simulink model "egk_new1"  (Simulink 7.5)
settings: Solver=ode45  StartTime=0.0  StopTime=0.1  RelTol=1e-3
libraries: powerlib x20, powerlib_extras x2
settings Model: Creator=Administrator  LastModifiedBy=Administrator

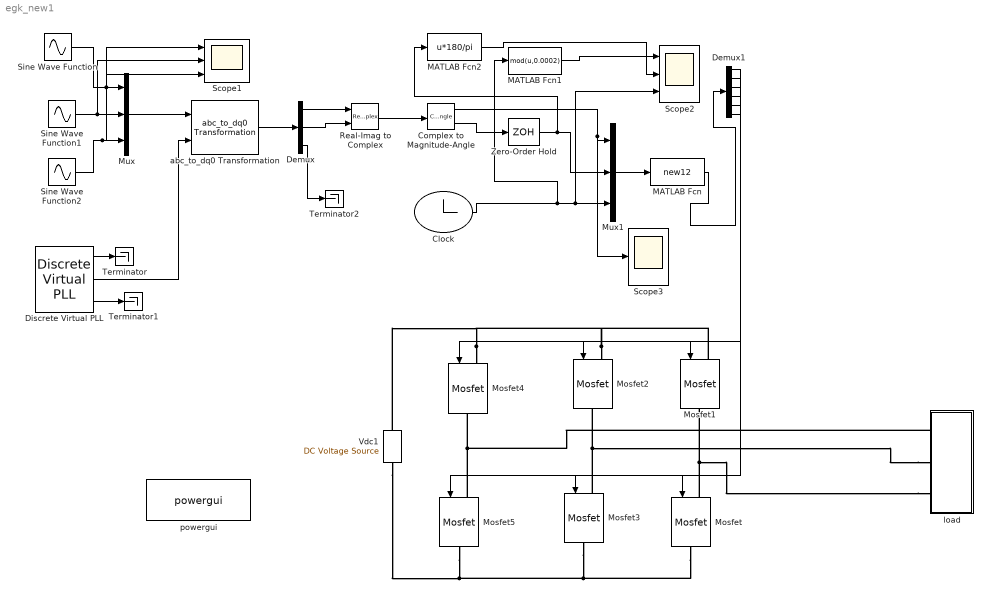
== system egk_new1 ==
  Clock : Clock
  Complex to Magnitude-Angle : ComplexToMagnitudeAngle  SampleTime=((2e-4)/8)/100
  Demux : Demux  Outputs=3
  Demux1 : Demux  Outputs=6
  Discrete Virtual PLL : powerlib_extras/Discrete  Control Blocks/Discrete Virtual PLL  DialogController=POWERSYS.PowerSysDialog  SystemSampleTime=-1  Freq=25  Phase=0  Ts=((2e-4)/8)/100
  MATLAB Fcn : MATLABFcn  MATLABFcn=new12  OutputDimensions=6  SampleTime=((2e-4)/8)/100
  MATLAB Fcn1 : MATLABFcn  MATLABFcn=mod(u,0.0002)  OutputDimensions=1
  MATLAB Fcn2 : MATLABFcn  MATLABFcn=u*180/pi  OutputDimensions=1
  Mosfet{,1..5} (6 alike) : powerlib/Power Electronics/Mosfet  DialogController=POWERSYS.PowerSysDialog  SystemSampleTime=-1  Ron=0.1  Lon=0  Rd=0.01  Vfd=0  IC=0  Rs=1e5  Cs=inf  Measurements=off
  Mux : Mux  Inputs=3
  Mux1 : Mux  Inputs=3
  Real-Imag to Complex : RealImagToComplex  SampleTime=((2e-4)/8)/100
  Scope1 : Scope  NumInputPorts=3
      settings: YMin=0~175~-217  YMax=42.5~200~-199
  Scope2 : Scope  NumInputPorts=3
      settings: YMin=0~-200~0.01975  YMax=0.0002~175~0.02175  SaveName=ScopeData2
  Scope3 : Scope
      settings: TimeRange=0.05  YMin=0.8164965808000001  YMax=0.8164965810500001
  Sine Wave Function : Sin  Amplitude=230  Bias=0  Frequency=2*pi*25  Phase=-pi/6  Samples=10  Offset=0
  Sine Wave Function1 : Sin  Amplitude=230  Bias=0  Frequency=2*pi*25  Phase=(2*pi/3)-(pi/6)  Samples=10  Offset=0
  Sine Wave Function2 : Sin  Amplitude=230  Bias=0  Frequency=2*pi*25  Phase=(4*pi/3)-(pi/6)  Samples=10  Offset=0
  Terminator : Terminator
  Terminator1 : Terminator
  Terminator2 : Terminator
  Vdc1 : powerlib/Electrical Sources/DC Voltage Source  DialogController=POWERSYS.PowerSysDialog  SystemSampleTime=-1  Amplitude=400  Measurements=None
  Zero-Order Hold : ZeroOrderHold  SampleTime=0.0001005
  abc_to_dq0 Transformation : powerlib_extras/Measurements/abc_to_dq0 Transformation  DialogController=POWERSYS.PowerSysDialog  SystemSampleTime=-1
  load : Subsystem
  powergui : powerlib/powergui  Priority=1  SystemSampleTime=-1  SimulationMode=Discrete  SampleTime=((2e-4)/8)/100  frequency=60  SPID=off  DisableSnubberDevices=off  DisableRonSwitches=off  DisableVfSwitches=off  SwTol=0  Interpol=off  frequencyindice=0  echomessages=off  HookPort=off  DisplayEquations=off  FunctionMessages=off  EnableUseOfTLC=off  x0status=blocks  RestoreLinks=warning  ResistiveCurrentMeasurement=off  Ylog=off  Xlog=on  ShowGrid=off  save=off  variable=ZData  structure=il  ZoomFFT=on  StartTime=0.025  cycles=2  DisplayStyle=1  fundamental=50  FreqAxis=on  MaxFrequency=500  frequencyindicesteady=1  RmsSteady=2  display=off  methode=off
  wires:
  Discrete Virtual PLL/1 -> Terminator/1
  Discrete Virtual PLL/3 -> Terminator1/1
  Sine Wave Function/1 -> Mux/1, Scope1/1
  Sine Wave Function1/1 -> Mux/2, Scope1/2
  Sine Wave Function2/1 -> Mux/3, Scope1/3
  Mux/1 -> abc_to_dq0 Transformation/1
  Discrete Virtual PLL/2 -> abc_to_dq0 Transformation/2
  abc_to_dq0 Transformation/1 -> Demux/1
  Demux/3 -> Terminator2/1
  Demux/1 -> Real-Imag to Complex/1
  Demux/2 -> Real-Imag to Complex/2
  Real-Imag to Complex/1 -> Complex to Magnitude-Angle/1
  Complex to Magnitude-Angle/2 -> Zero-Order Hold/1
  Complex to Magnitude-Angle/1 -> Mux1/1, Scope3/1
  Zero-Order Hold/1 -> Mux1/2, MATLAB Fcn2/1
  Mux1/1 -> MATLAB Fcn/1
  Clock/1 -> MATLAB Fcn1/1, Mux1/3, Scope2/3
  MATLAB Fcn1/1 -> Scope2/1
  MATLAB Fcn2/1 -> Scope2/2
  MATLAB Fcn/1 -> Demux1/1
  Demux1/1 -> Mosfet4/1
  Demux1/2 -> Mosfet5/1
  Demux1/3 -> Mosfet2/1
  Demux1/4 -> Mosfet3/1
  Demux1/5 -> Mosfet1/1
  Demux1/6 -> Mosfet/1
  connections:
  Mosfet2/LConn1 -- Mosfet1/LConn1 -- Mosfet4/LConn1 -- Vdc1/RConn1
  load/LConn1 -- Mosfet5/LConn1 -- Mosfet4/RConn1
  Mosfet3/RConn1 -- Mosfet/RConn1 -- Vdc1/LConn1 -- Mosfet5/RConn1
  load/LConn2 -- Mosfet3/LConn1 -- Mosfet2/RConn1
  load/LConn3 -- Mosfet/LConn1 -- Mosfet1/RConn1

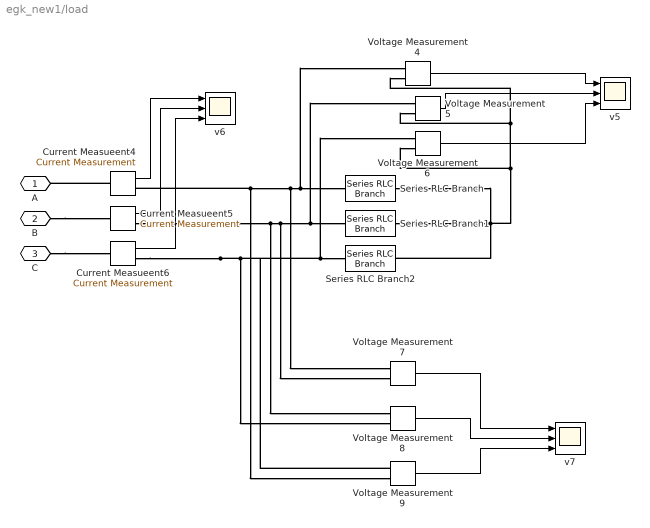
== system egk_new1/load ==
  Current Measueent4 : powerlib/Measurements/Current Measurement  DialogController=POWERSYS.PowerSysDialog  SystemSampleTime=-1  PhasorSimulation=off  OutputType=Complex  PSBequivalent=0
  Current Measueent5 : powerlib/Measurements/Current Measurement  DialogController=POWERSYS.PowerSysDialog  SystemSampleTime=-1  PhasorSimulation=off  OutputType=Complex  PSBequivalent=0
  Current Measueent6 : powerlib/Measurements/Current Measurement  DialogController=POWERSYS.PowerSysDialog  SystemSampleTime=-1  PhasorSimulation=off  OutputType=Complex  PSBequivalent=0
  Series RLC Branch : powerlib/Elements/Series RLC Branch  DialogController=POWERSYS.PowerSysDialog  PhysicalDomain=powersysdomain  SubClassName=unknown  LeftPortType=p1  RightPortType=p1  LConnTagsString=__new0  RConnTagsString=__new0  BranchType=R  Resistance=100  Inductance=40e-3  SetiL0=off  InitialCurrent=0  Capacitance=1e-6  Setx0=off  InitialVoltage=0  Measurements=Branch voltage and current
  Series RLC Branch1 : powerlib/Elements/Series RLC Branch  DialogController=POWERSYS.PowerSysDialog  PhysicalDomain=powersysdomain  SubClassName=unknown  LeftPortType=p1  RightPortType=p1  LConnTagsString=__new0  RConnTagsString=__new0  BranchType=R  Resistance=100  Inductance=40e-3  SetiL0=off  InitialCurrent=0  Capacitance=1e-6  Setx0=off  InitialVoltage=0  Measurements=Branch voltage and current
  Series RLC Branch2 : powerlib/Elements/Series RLC Branch  DialogController=POWERSYS.PowerSysDialog  PhysicalDomain=powersysdomain  SubClassName=unknown  LeftPortType=p1  RightPortType=p1  LConnTagsString=__new0  RConnTagsString=__new0  BranchType=R  Resistance=100  Inductance=40e-3  SetiL0=off  InitialCurrent=0  Capacitance=1e-6  Setx0=off  InitialVoltage=0  Measurements=Branch voltage and current
  Voltage Measurement{4..9} (6 alike) : powerlib/Measurements/Voltage Measurement  DialogController=POWERSYS.PowerSysDialog  SystemSampleTime=-1  PhasorSimulation=off  OutputType=Complex  PSBequivalent=0
  v5 : Scope  NumInputPorts=3
      settings: TimeRange=0.1  YMin=-300~-300~-300  YMax=300~300~300  SaveName=phase_v  MaxDataPoints=5000000
  v6 : Scope  NumInputPorts=3
      settings: YMin=-25~-5~-5  YMax=275~5~5  SaveName=il  MaxDataPoints=5000000
  v7 : Scope  NumInputPorts=3
      settings: YMin=-25~-5~-5  YMax=275~5~5  SaveName=line_v  MaxDataPoints=5000000
  A : PMIOPort  Port=1  Side=Left
  B : PMIOPort  Port=2  Side=Left
  C : PMIOPort  Port=3  Side=Left
  wires:
  Voltage Measurement4/1 -> v5/1
  Voltage Measurement5/1 -> v5/2
  Voltage Measurement6/1 -> v5/3
  Current Measueent4/1 -> v6/1
  Current Measueent5/1 -> v6/2
  Current Measueent6/1 -> v6/3
  Voltage Measurement7/1 -> v7/1
  Voltage Measurement8/1 -> v7/2
  Voltage Measurement9/1 -> v7/3
  connections:
  Voltage Measurement5/LConn2 -- Voltage Measurement4/LConn2 -- Voltage Measurement6/LConn2 -- Series RLC Branch2/RConn1 -- Series RLC Branch1/RConn1 -- Series RLC Branch/RConn1
  Current Measueent4/LConn1 -- A/RConn1
  Current Measueent4/RConn1 -- Series RLC Branch/LConn1 -- Voltage Measurement4/LConn1 -- Voltage Measurement7/LConn1 -- Voltage Measurement9/LConn2
  B/RConn1 -- Current Measueent5/LConn1
  Current Measueent5/RConn1 -- Series RLC Branch1/LConn1 -- Voltage Measurement5/LConn1 -- Voltage Measurement7/LConn2 -- Voltage Measurement8/LConn1
  C/RConn1 -- Current Measueent6/LConn1
  Current Measueent6/RConn1 -- Voltage Measurement9/LConn1 -- Series RLC Branch2/LConn1 -- Voltage Measurement6/LConn1 -- Voltage Measurement8/LConn2
